simulink model "PID_controller_lat_stage4_plot"  (R2019a)
settings: Solver=VariableStepAuto  StartTime=0.0  StopTime=100  FixedStep=1e-4  RelTol=1e-5
undefined symbols (not defined in the file): geometry, sys
libraries: simulink x3, aerolibactuator x2
settings Model: Creator=tyson  LastModifiedBy=tyson
settings DebuggingCC: TimeAdjustmentMsg=warning

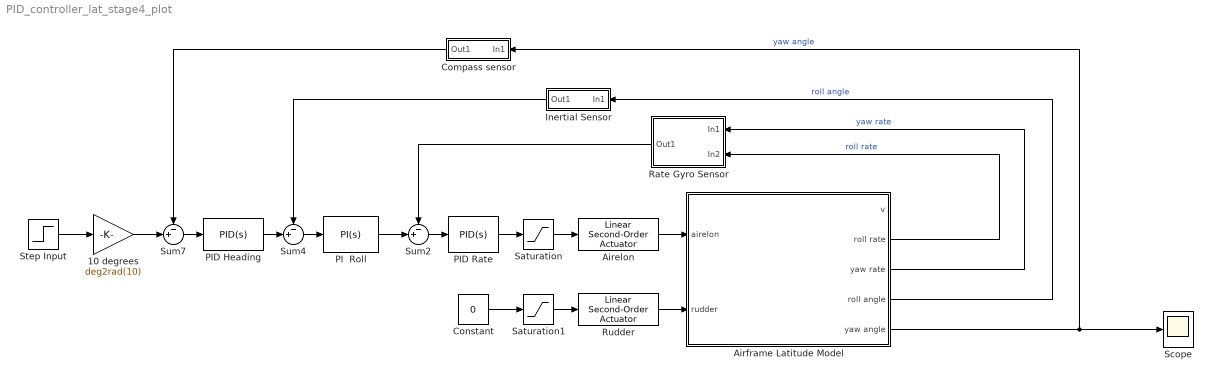
== system PID_controller_lat_stage4_plot ==
  10 degrees : Gain  Gain=deg2rad(10)
  Airelon : aerolibactuator/Linear Second-Order Actuator  wn_fin=actuators.naturalFreq  z_fin=actuators.dampingRatio  fin_act_0=0  fin_act_vel=0
      settings: SourceProductName=Aerospace Blockset  SourceProductBaseCode=AE
  Airframe Latitude Model : Subsystem
      mask Display: image('/home/tyson/Dropbox/Academic/4th Year/ELEN4011/matlab/icons/airframe_lat.png');
  Compass sensor : Subsystem
  Constant : Constant  Value=0
  Inertial Sensor : Subsystem
  PI  Roll : simulink/Continuous/PID Controller  Controller=PI  Form=Parallel  TimeDomain=Continuous-time  SampleTime=-1  IntegratorMethod=Forward Euler  FilterMethod=Forward Euler  ControllerParametersSource=internal  P=13.8346091340675  I=2.4410545354894  D=0  UseFilter=on  N=100  TunerSelectOption=Transfer Function Based (PID Tuner App)  InitialConditionSource=internal  InitialConditionForIntegrator=0  InitialConditionForFilter=0  DifferentiatorICPrevScaledInput=0  ExternalReset=none  TrackingMode=off  Kt=1  LimitOutput=on  UpperSaturationLimit=geometry.airelon.limits(1)  LowerSaturationLimit=geometry.airelon.limits(2)  LinearizeAsGain=on  AntiWindupMode=clamping  Kb=1  POutMin=[]  POutMax=[]  IOutMin=[]  IOutMax=[]  DOutMin=[]  DOutMax=[]  NOutMin=[]  NOutMax=[]  SumOutMin=[]  SumOutMax=[]  SaturationOutMin=[]  SaturationOutMax=[]  PParamMin=[]  PParamMax=[]  IParamMin=[]  IParamMax=[]  DParamMin=[]  DParamMax=[]  NParamMin=[]  NParamMax=[]  KbParamMin=[]  KbParamMax=[]  KtParamMin=[]  KtParamMax=[]  KbOutMin=[]  KbOutMax=[]  KtOutMin=[]  KtOutMax=[]  IntegratorOutMin=[]  IntegratorOutMax=[]  FilterOutMin=[]  FilterOutMax=[]  SumI1OutMin=[]  SumI1OutMax=[]  SumI2OutMin=[]  SumI2OutMax=[]  SumI3OutMin=[]  SumI3OutMax=[]  SumI4OutMin=[]  SumI4OutMax=[]  SumDOutMin=[]  SumDOutMax=[]  DifferentiatorOutMin=[]  DifferentiatorOutMax=[]  FilterDiffOutCoefMin=[]  FilterDiffOutCoefMax=[]  ReciprocalOutMin=[]  ReciprocalOutMax=[]  SumDenOutMin=[]  SumDenOutMax=[]  SumNumOutMin=[]  SumNumOutMax=[]  DivideOutMin=[]  DivideOutMax=[]  IntegratorContinuousStateAttributes=''  IntegratorStateMustResolveToSignalObject=off  IntegratorRTWStateStorageClass=Auto  FilterContinuousStateAttributes=''  FilterStateMustResolveToSignalObject=off  FilterRTWStateStorageClass=Auto  ParallelPVariant=InternalParameters  IdealPVariant=Disabled  IVariant=InternalParameters  DVariant=Disabled  IntegratorVariant=Continuous  SatVariant=Enabled  AWVariant=ContClampingParallel  PCopyVariant=Disabled  TRVariant=Disabled  FdbkBlocksVariant=Forward  IdealPFdbkVariant=Disabled  SatFdbkVariant=Disabled  DerivativeFilterVariant=Disabled  NVariant=Disabled  NCopyVariant=Disabled_SignalSpec  FilterICVariant=Disabled  IntegratorICVariant=InternalICs  ExternalResetVariant=Disabled  TRSumVariant=Passthrough  SumFdbkVariant=Disabled  SumVariant=Sum_PI
  PID Heading : simulink/Continuous/PID Controller  Controller=PID  Form=Parallel  TimeDomain=Continuous-time  SampleTime=-1  IntegratorMethod=Forward Euler  FilterMethod=Forward Euler  ControllerParametersSource=internal  P=0.897329069683847  I=0.0028476992795986  D=-0.236062607776474  UseFilter=on  N=3.80123340217236  TunerSelectOption=Transfer Function Based (PID Tuner App)  InitialConditionSource=internal  InitialConditionForIntegrator=0  InitialConditionForFilter=0  DifferentiatorICPrevScaledInput=0  ExternalReset=none  TrackingMode=off  Kt=1  LimitOutput=on  UpperSaturationLimit=pi  LowerSaturationLimit=-pi  LinearizeAsGain=on  AntiWindupMode=clamping  Kb=1  POutMin=[]  POutMax=[]  IOutMin=[]  IOutMax=[]  DOutMin=[]  DOutMax=[]  NOutMin=[]  NOutMax=[]  SumOutMin=[]  SumOutMax=[]  SaturationOutMin=[]  SaturationOutMax=[]  PParamMin=[]  PParamMax=[]  IParamMin=[]  IParamMax=[]  DParamMin=[]  DParamMax=[]  NParamMin=[]  NParamMax=[]  KbParamMin=[]  KbParamMax=[]  KtParamMin=[]  KtParamMax=[]  KbOutMin=[]  KbOutMax=[]  KtOutMin=[]  KtOutMax=[]  IntegratorOutMin=[]  IntegratorOutMax=[]  FilterOutMin=[]  FilterOutMax=[]  SumI1OutMin=[]  SumI1OutMax=[]  SumI2OutMin=[]  SumI2OutMax=[]  SumI3OutMin=[]  SumI3OutMax=[]  SumI4OutMin=[]  SumI4OutMax=[]  SumDOutMin=[]  SumDOutMax=[]  DifferentiatorOutMin=[]  DifferentiatorOutMax=[]  FilterDiffOutCoefMin=[]  FilterDiffOutCoefMax=[]  ReciprocalOutMin=[]  ReciprocalOutMax=[]  SumDenOutMin=[]  SumDenOutMax=[]  SumNumOutMin=[]  SumNumOutMax=[]  DivideOutMin=[]  DivideOutMax=[]  IntegratorContinuousStateAttributes=''  IntegratorStateMustResolveToSignalObject=off  IntegratorRTWStateStorageClass=Auto  FilterContinuousStateAttributes=''  FilterStateMustResolveToSignalObject=off  FilterRTWStateStorageClass=Auto  ParallelPVariant=InternalParameters  IdealPVariant=Disabled  IVariant=InternalParameters  DVariant=InternalParameters  IntegratorVariant=Continuous  SatVariant=Enabled  AWVariant=ContClampingParallel  PCopyVariant=Disabled  TRVariant=Disabled  FdbkBlocksVariant=Forward  IdealPFdbkVariant=Disabled  SatFdbkVariant=Disabled  DerivativeFilterVariant=ContFilter  NVariant=InternalParameters  NCopyVariant=Disabled  FilterICVariant=InternalICsFilter  IntegratorICVariant=InternalICs  ExternalResetVariant=Disabled  TRSumVariant=Passthrough  SumFdbkVariant=Disabled  SumVariant=Sum_PID
  PID Rate : simulink/Continuous/PID Controller  Controller=PID  Form=Parallel  TimeDomain=Continuous-time  SampleTime=-1  IntegratorMethod=Forward Euler  FilterMethod=Forward Euler  ControllerParametersSource=internal  P=0.590153901924478  I=1.57249325880203  D=0.0263005887519142  UseFilter=on  N=1926.62602358078  TunerSelectOption=Transfer Function Based (PID Tuner App)  InitialConditionSource=internal  InitialConditionForIntegrator=0  InitialConditionForFilter=0  DifferentiatorICPrevScaledInput=0  ExternalReset=none  TrackingMode=off  Kt=1  LimitOutput=on  UpperSaturationLimit=pi  LowerSaturationLimit=-pi  LinearizeAsGain=on  AntiWindupMode=clamping  Kb=1  POutMin=[]  POutMax=[]  IOutMin=[]  IOutMax=[]  DOutMin=[]  DOutMax=[]  NOutMin=[]  NOutMax=[]  SumOutMin=[]  SumOutMax=[]  SaturationOutMin=[]  SaturationOutMax=[]  PParamMin=[]  PParamMax=[]  IParamMin=[]  IParamMax=[]  DParamMin=[]  DParamMax=[]  NParamMin=[]  NParamMax=[]  KbParamMin=[]  KbParamMax=[]  KtParamMin=[]  KtParamMax=[]  KbOutMin=[]  KbOutMax=[]  KtOutMin=[]  KtOutMax=[]  IntegratorOutMin=[]  IntegratorOutMax=[]  FilterOutMin=[]  FilterOutMax=[]  SumI1OutMin=[]  SumI1OutMax=[]  SumI2OutMin=[]  SumI2OutMax=[]  SumI3OutMin=[]  SumI3OutMax=[]  SumI4OutMin=[]  SumI4OutMax=[]  SumDOutMin=[]  SumDOutMax=[]  DifferentiatorOutMin=[]  DifferentiatorOutMax=[]  FilterDiffOutCoefMin=[]  FilterDiffOutCoefMax=[]  ReciprocalOutMin=[]  ReciprocalOutMax=[]  SumDenOutMin=[]  SumDenOutMax=[]  SumNumOutMin=[]  SumNumOutMax=[]  DivideOutMin=[]  DivideOutMax=[]  IntegratorContinuousStateAttributes=''  IntegratorStateMustResolveToSignalObject=off  IntegratorRTWStateStorageClass=Auto  FilterContinuousStateAttributes=''  FilterStateMustResolveToSignalObject=off  FilterRTWStateStorageClass=Auto  ParallelPVariant=InternalParameters  IdealPVariant=Disabled  IVariant=InternalParameters  DVariant=InternalParameters  IntegratorVariant=Continuous  SatVariant=Enabled  AWVariant=ContClampingParallel  PCopyVariant=Disabled  TRVariant=Disabled  FdbkBlocksVariant=Forward  IdealPFdbkVariant=Disabled  SatFdbkVariant=Disabled  DerivativeFilterVariant=ContFilter  NVariant=InternalParameters  NCopyVariant=Disabled  FilterICVariant=InternalICsFilter  IntegratorICVariant=InternalICs  ExternalResetVariant=Disabled  TRSumVariant=Passthrough  SumFdbkVariant=Disabled  SumVariant=Sum_PID
  Rate Gyro Sensor : Subsystem
  Rudder : aerolibactuator/Linear Second-Order Actuator  wn_fin=actuators.naturalFreq  z_fin=actuators.dampingRatio  fin_act_0=0  fin_act_vel=0
      settings: SourceProductName=Aerospace Blockset  SourceProductBaseCode=AE
  Saturation : Saturate  UpperLimit=geometry.airelon.limits(1)  LowerLimit=geometry.airelon.limits(2)  LinearizeAsGain=off
  Saturation1 : Saturate  UpperLimit=geometry.rudder.limits(1)  LowerLimit=geometry.rudder.limits(2)  LinearizeAsGain=off
  Scope : Scope
  Step Input : Step
  Sum2 : Sum  Inputs=-+|
  Sum4 : Sum  Inputs=-+|
  Sum7 : Sum  Inputs=-+|
  wires:
  Step Input/1 -> 10 degrees/1
  Airframe Latitude Model/5(yaw angle) -> Compass sensor/1(In1), Scope/1  "yaw angle"
  Sum7/1 -> PID Heading/1
  Airframe Latitude Model/3(yaw rate) -> Rate Gyro Sensor/1(In1)  "yaw rate"
  Airframe Latitude Model/2(roll rate) -> Rate Gyro Sensor/2(In2)  "roll rate"
  Airelon/1 -> Airframe Latitude Model/1(airelon)
  Airframe Latitude Model/4(roll angle) -> Inertial Sensor/1(In1)  "roll angle"
  Saturation/1 -> Airelon/1
  PI  Roll/1 -> Sum2/2
  Sum4/1 -> PI  Roll/1
  Rate Gyro Sensor/1(Out1) -> Sum2/1
  Inertial Sensor/1(Out1) -> Sum4/1
  Constant/1 -> Saturation1/1
  PID Heading/1 -> Sum4/2
  Rudder/1 -> Airframe Latitude Model/2(rudder)
  Sum2/1 -> PID Rate/1
  Compass sensor/1(Out1) -> Sum7/1
  10 degrees/1 -> Sum7/2
  PID Rate/1 -> Saturation/1
  Saturation1/1 -> Rudder/1

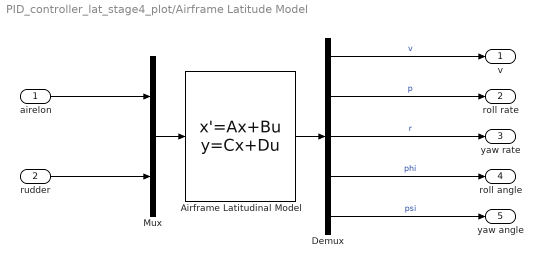
== system PID_controller_lat_stage4_plot/Airframe Latitude Model ==
  airelon : Inport
  rudder : Inport  Port=2
  Airframe Latitudinal Model : StateSpace  A=sys.lat.A  B=sys.lat.B  C=sys.lat.C  D=sys.lat.D  InitialCondition=0
  Demux : Demux  Outputs=5
  Mux : Mux  Inputs=2
  v : Outport
  roll rate : Outport  Port=2
  yaw rate : Outport  Port=3
  roll angle : Outport  Port=4
  yaw angle : Outport  Port=5
  wires:
  rudder/1 -> Mux/2
  Demux/4 -> roll angle/1  "phi"
  Demux/3 -> yaw rate/1  "r"
  Mux/1 -> Airframe Latitudinal Model/1
  Airframe Latitudinal Model/1 -> Demux/1
  Demux/1 -> v/1  "v"
  Demux/2 -> roll rate/1  "p"
  Demux/5 -> yaw angle/1  "psi"
  airelon/1 -> Mux/1

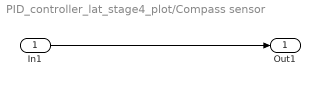
== system PID_controller_lat_stage4_plot/Compass sensor ==
  In1 : Inport
  Out1 : Outport
  wires:
  In1/1 -> Out1/1

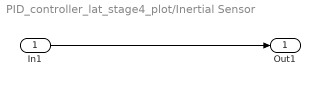
== system PID_controller_lat_stage4_plot/Inertial Sensor ==
  In1 : Inport
  Out1 : Outport
  wires:
  In1/1 -> Out1/1

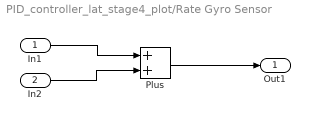
== system PID_controller_lat_stage4_plot/Rate Gyro Sensor ==
  In1 : Inport
  In2 : Inport  Port=2
  Plus : Sum
  Out1 : Outport
  wires:
  In1/1 -> Plus/1
  In2/1 -> Plus/2
  Plus/1 -> Out1/1
